simulink model "ZOH"  (R2021a)
settings: Solver=VariableStepAuto  StartTime=0.0  StopTime=20  RelTol=1e-3
libraries: robotlib x17, simulink_extras x1
settings Model: EnablePacing=on  Creator=chnwa  LastModifiedBy=chnwa

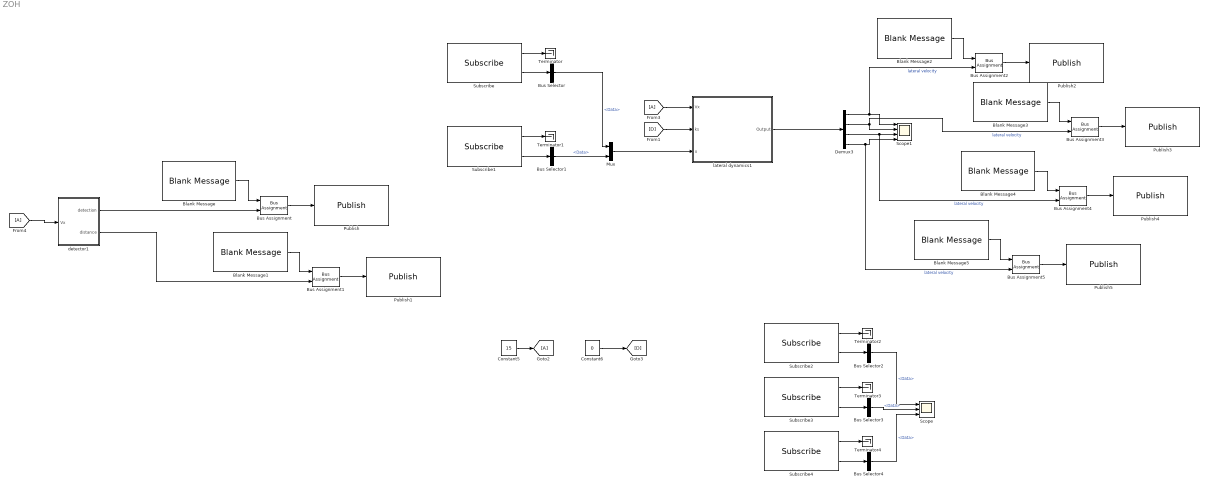
== system ZOH ==
  Blank Message{,1..5} (6 alike) : robotlib/Blank Message  messageClass=Message  entityType=std_msgs/Float64  messageType=std_msgs/Float64  SampleTime=inf  legacyBusStruct=off
  Bus Assignment{,1..5} (6 alike) : BusAssignment  AssignedSignals=Data
  Bus Selector{,1..4} (5 alike) : BusSelector  OutputSignals=Data
  Constant5 : Constant  Value=15
  Constant6 : Constant  Value=0
  Demux3 : Demux
  Mux : Mux  Inputs=2
  Publish : robotlib/Publish  topicSource=Specify your own  topic=/Detection  messageType=std_msgs/Float64  legacyBusStruct=off  messageQueueLength=1
  Publish1 : robotlib/Publish  topicSource=Specify your own  topic=/Distance  messageType=std_msgs/Float64  legacyBusStruct=off  messageQueueLength=1
  Publish2 : robotlib/Publish  topicSource=Specify your own  topic=/States1  messageType=std_msgs/Float64  legacyBusStruct=off  messageQueueLength=1
  Publish3 : robotlib/Publish  topicSource=Specify your own  topic=/States2  messageType=std_msgs/Float64  legacyBusStruct=off  messageQueueLength=1
  Publish4 : robotlib/Publish  topicSource=Specify your own  topic=/States3  messageType=std_msgs/Float64  legacyBusStruct=off  messageQueueLength=1
  Publish5 : robotlib/Publish  topicSource=Specify your own  topic=/States4  messageType=std_msgs/Float64  legacyBusStruct=off  messageQueueLength=1
  Scope : Scope  NumInputPorts=3
  Scope1 : Scope  NumInputPorts=4
  Subscribe : robotlib/Subscribe  topicSource=Specify your own  topic=/Mv1  messageType=std_msgs/Float64  SampleTime=-1  legacyBusStruct=off  messageQueueLength=1
  Subscribe1 : robotlib/Subscribe  topicSource=Specify your own  topic=/Mv2  messageType=std_msgs/Float64  SampleTime=-1  legacyBusStruct=off  messageQueueLength=1
  Subscribe2 : robotlib/Subscribe  topicSource=Specify your own  topic=/Cost  messageType=std_msgs/Float64  SampleTime=-1  legacyBusStruct=off  messageQueueLength=1
  Subscribe3 : robotlib/Subscribe  topicSource=Specify your own  topic=/Flag  messageType=std_msgs/Float64  SampleTime=-1  legacyBusStruct=off  messageQueueLength=1
  Subscribe4 : robotlib/Subscribe  topicSource=Specify your own  topic=/Time  messageType=std_msgs/Float64  SampleTime=-1  legacyBusStruct=off  messageQueueLength=1
  Terminator{,1..4} (5 alike) : Terminator
  detector1 : Subsystem
  lateral dynamics1 : Subsystem
  wires:
  [D] -> lateral dynamics1/2(ks)
  Mux/1 -> lateral dynamics1/3(u)
  Demux3/1 -> Bus Assignment2/2, Scope1/1  "lateral velocity"
  detector1/1(detection) -> Bus Assignment/2
  Constant5/1 -> [A]
  [A] -> detector1/1(Vx)
  Constant6/1 -> [D]
  lateral dynamics1/1(Output) -> Demux3/1
  [A] -> lateral dynamics1/1(Vx)
  Subscribe/2 -> Bus Selector/1
  Subscribe/1 -> Terminator/1
  Bus Selector/1 -> Mux/1  "<Data>"
  Subscribe1/2 -> Bus Selector1/1
  Subscribe1/1 -> Terminator1/1
  Bus Selector1/1 -> Mux/2  "<Data>"
  Blank Message/1 -> Bus Assignment/1
  Bus Assignment/1 -> Publish/1
  Blank Message1/1 -> Bus Assignment1/1
  detector1/2(distance) -> Bus Assignment1/2
  Bus Assignment1/1 -> Publish1/1
  Blank Message2/1 -> Bus Assignment2/1
  Bus Assignment2/1 -> Publish2/1
  Bus Assignment3/1 -> Publish3/1
  Blank Message3/1 -> Bus Assignment3/1
  Demux3/2 -> Bus Assignment3/2, Scope1/2  "lateral velocity"
  Bus Assignment4/1 -> Publish4/1
  Blank Message4/1 -> Bus Assignment4/1
  Demux3/3 -> Bus Assignment4/2, Scope1/3  "lateral velocity"
  Bus Assignment5/1 -> Publish5/1
  Blank Message5/1 -> Bus Assignment5/1
  Demux3/4 -> Bus Assignment5/2, Scope1/4  "lateral velocity"
  Subscribe2/2 -> Bus Selector2/1
  Subscribe2/1 -> Terminator2/1
  Subscribe3/2 -> Bus Selector3/1
  Subscribe3/1 -> Terminator3/1
  Subscribe4/1 -> Terminator4/1
  Subscribe4/2 -> Bus Selector4/1
  Bus Selector2/1 -> Scope/1  "<Data>"
  Bus Selector3/1 -> Scope/2  "<Data>"
  Bus Selector4/1 -> Scope/3  "<Data>"

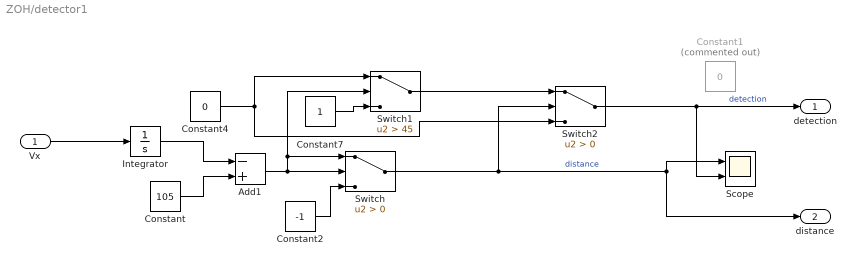
== system ZOH/detector1 ==
  Vx : Inport
  Add1 : Sum  Inputs=-+
  Constant : Constant  Value=105
  Constant1 : Constant  Commented=on  Value=0
  Constant2 : Constant  Value=-1
  Constant4 : Constant  Value=0
  Constant7 : Constant
  Integrator : Integrator
  Scope : Scope  NumInputPorts=2
  Switch : Switch  Criteria=u2 > Threshold
  Switch1 : Switch  Criteria=u2 > Threshold  Threshold=45
  Switch2 : Switch  Criteria=u2 > Threshold
  detection : Outport
  distance : Outport  Port=2
  wires:
  Constant2/1 -> Switch/3
  Constant4/1 -> Switch2/3, Switch1/1
  Vx/1 -> Integrator/1
  Integrator/1 -> Add1/1
  Switch/1 -> Switch2/2, distance/1, Scope/1  "distance"
  Constant7/1 -> Switch1/3
  Add1/1 -> Switch1/2, Switch/1, Switch/2
  Switch1/1 -> Switch2/1
  Constant/1 -> Add1/2
  Switch2/1 -> detection/1, Scope/2  "detection"

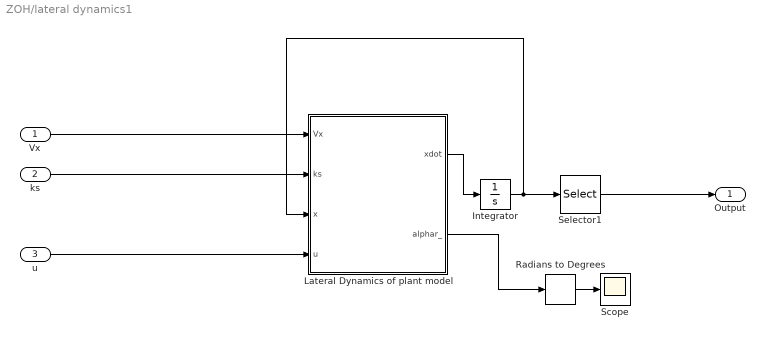
== system ZOH/lateral dynamics1 ==
  Vx : Inport
  ks : Inport  Port=2
  u : Inport  Port=3
  Integrator : Integrator
  Lateral Dynamics of plant model : MATLAB Function  TreatAsAtomicUnit=on
  Radians to Degrees : simulink_extras/Transformations/Radians to Degrees
  Scope : Scope
  Selector1 : Selector  InputPortWidth=4  IndexOptions=Index vector (dialog)  Indices=[1 2 3 4]  OutputSizes=1
  Output : Outport
  wires:
  u/1 -> Lateral Dynamics of plant model/4(u)
  Lateral Dynamics of plant model/1(xdot) -> Integrator/1
  Integrator/1 -> Selector1/1, Lateral Dynamics of plant model/3(x)
  Selector1/1 -> Output/1
  ks/1 -> Lateral Dynamics of plant model/2(ks)
  Vx/1 -> Lateral Dynamics of plant model/1(Vx)
  Lateral Dynamics of plant model/2(alphar_) -> Radians to Degrees/1
  Radians to Degrees/1 -> Scope/1

== matlab function ZOH/lateral dynamics1/Lateral Dynamics of plant model ==
  data: Vx input; ks input; x input; u input; xdot output; alphar_ output
function [xdot,alphar_] = fcn(Vx,ks, x, u)

%Plant Model parameters
m = 2272;   %mass
Iz = 4600;  %rotational inertia
lf = 1.11;  % distance from front axle to the mass center
lr = 1.67;  % distance from rear axle to the mass center
C_a = 1.822e5; % rear cornering stifness 

%Enviroment parameters
miu = 0.7; %frction cooeficient 0.7 for dry road and 0.4 for wet
g = 9.81; % gravity

Fz = m*g*lf/(lf+lr); % the load that beared by the rear tire

%calculate alpha
Vy = x(1); %lateral velocity
r = x(2);  %yaw rate
alphar_ = Vy/Vx-lr*r/Vx;   %calculate linearzing point

%tire model
threshold = atan(3*miu*Fz/C_a);
if abs(alphar_)<threshold
    Fyr_ = -C_a*tan(alphar_)+C_a^2/(3*miu*Fz)*abs(tan(alphar_))*tan(alphar_)-C_a^3/(27*miu^2*Fz^2)*tan(alphar_)^3;
    if alphar_>= 0
        Cr_ = -C_a*sec(alphar_)^2+C_a^2/(3*miu*Fz)*(2*sec(alphar_)^2*tan(alphar_))-C_a^3/(27*miu^2*Fz^2)*(3*tan(alphar_)^2*sec(alphar_)^2);
    else
        Cr_ = -C_a*sec(alphar_)^2-C_a^2/(3*miu*Fz)*(2*sec(alphar_)^2*tan(alphar_))-C_a^3/(27*miu^2*Fz^2)*(3*tan(alphar_)^2*sec(alphar_)^2);
    end
else
    Fyr_ = -miu*Fz*sign(alphar_);
    Cr_ = 0;
end

%Continuous-time model
Ac = [Cr_/(m*Vx) -lr*Cr_/(m*Vx)-Vx 0 0;
    -lr*Cr_/(Iz*Vx) lr^2*Cr_/(Iz*Vx) 0 0;
    0 1 0 0;
    1 0 Vx 0];
Bc = [1/m 0;
    lf/Iz 1/Iz;
    0 0;
    0 0];
dcc = [(Fyr_-Cr_*alphar_)/m;
    -lr*(Fyr_-Cr_*alphar_)/Iz;
    -Vx*ks;
    0];

% Cc =eye(4);
% Dc =zeros(4,2);
xdot = Ac*x + Bc*u +dcc;
% y = C*x + D*u;
